simulink model "tf_hex"  (R2020a)
settings: Solver=FixedStepAuto  StartTime=0.0  StopTime=10.0  FixedStep=step_size  RelTol=1e-3
values from neighbouring files (symbols this model uses):
  A = diag([Ax Ax Ax])    [tf_model_sim.m]
  g = 9.81    [tf_model_sim.m]
  m = 1.89    [tf_model_sim.m]
  pitch_tf = tf([omega_n^2], [1 2*zeta*omega_n omega_n^2])*tf([pl],[1 pl],'InputDelay',0.09)    [tf_model_sim.m]
  Ts = 0.01    [tf_model_sim.m]
settings Model: Creator=pala  LastModifiedBy=pala
settings DataIOCC: SaveFormat=StructureWithTime  ReturnWorkspaceOutputs=off

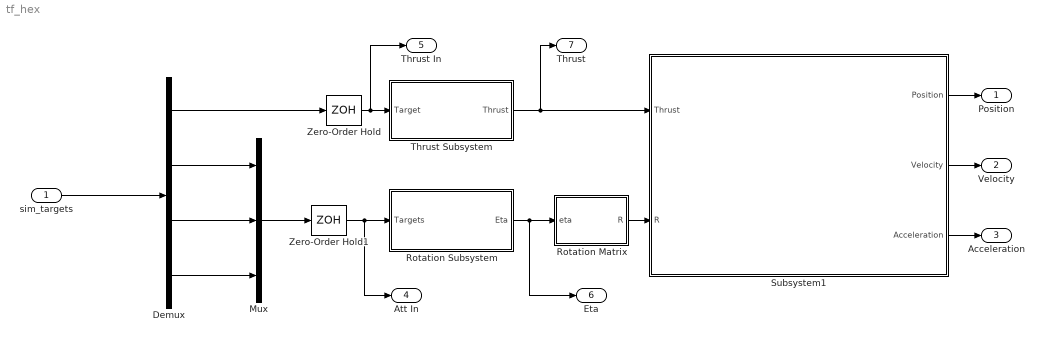
== system tf_hex ==
  sim_targets : Inport
  Demux : Demux
  Mux : Mux  Inputs=3
  Rotation Matrix : MATLAB Function  TreatAsAtomicUnit=on
  Rotation Subsystem : Subsystem
  Subsystem1 : Subsystem
  Thrust Subsystem : Subsystem
  Zero-Order Hold : ZeroOrderHold  SampleTime=Ts
  Zero-Order Hold1 : ZeroOrderHold  SampleTime=Ts
  Position : Outport
  Velocity : Outport  Port=2
  Acceleration : Outport  Port=3
  Att In : Outport  Port=4
  Thrust In : Outport  Port=5
  Eta : Outport  Port=6
  Thrust : Outport  Port=7
  wires:
  sim_targets/1 -> Demux/1
  Demux/2 -> Mux/1
  Demux/3 -> Mux/2
  Demux/4 -> Mux/3
  Subsystem1/2(Velocity) -> Velocity/1
  Subsystem1/3(Acceleration) -> Acceleration/1
  Thrust Subsystem/1(Thrust) -> Thrust/1, Subsystem1/1(Thrust)
  Subsystem1/1(Position) -> Position/1
  Rotation Matrix/1(R) -> Subsystem1/2(R)
  Zero-Order Hold/1 -> Thrust In/1, Thrust Subsystem/1(Target)
  Demux/1 -> Zero-Order Hold/1
  Mux/1 -> Zero-Order Hold1/1
  Zero-Order Hold1/1 -> Att In/1, Rotation Subsystem/1(Targets)
  Rotation Subsystem/1(Eta) -> Eta/1, Rotation Matrix/1(eta)

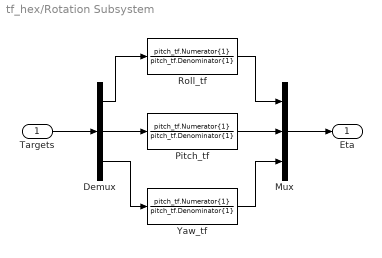
== system tf_hex/Rotation Subsystem ==
  Targets : Inport
  Demux : Demux  Outputs=3
  Mux : Mux  Inputs=3
  Pitch_tf : TransferFcn  Numerator=pitch_tf.Numerator{1}  Denominator=pitch_tf.Denominator{1}
  Roll_tf : TransferFcn  Numerator=pitch_tf.Numerator{1}  Denominator=pitch_tf.Denominator{1}
  Yaw_tf : TransferFcn  Numerator=pitch_tf.Numerator{1}  Denominator=pitch_tf.Denominator{1}
  Eta : Outport
  wires:
  Demux/1 -> Roll_tf/1
  Demux/2 -> Pitch_tf/1
  Demux/3 -> Yaw_tf/1
  Targets/1 -> Demux/1
  Pitch_tf/1 -> Mux/2
  Roll_tf/1 -> Mux/1
  Yaw_tf/1 -> Mux/3
  Mux/1 -> Eta/1

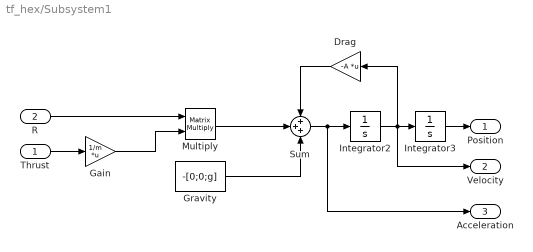
== system tf_hex/Subsystem1 ==
  Thrust : Inport
  R : Inport  Port=2
  Drag : Gain  Gain=-A  Multiplication=Matrix(K*u)
  Gain : Gain  Gain=1/m  Multiplication=Matrix(K*u)
  Gravity : Constant  Value=-[0;0;g]
  Integrator2 : Integrator
  Integrator3 : Integrator
  Multiply : Product  Inputs=**  Multiplication=Matrix(*)
  Sum : Sum  Inputs=+++
  Position : Outport  VectorParamsAs1DForOutWhenUnconnected=off
  Velocity : Outport  Port=2  VectorParamsAs1DForOutWhenUnconnected=off
  Acceleration : Outport  Port=3  VectorParamsAs1DForOutWhenUnconnected=off
  wires:
  Sum/1 -> Acceleration/1, Integrator2/1
  R/1 -> Multiply/1
  Gravity/1 -> Sum/3
  Thrust/1 -> Gain/1
  Integrator3/1 -> Position/1
  Integrator2/1 -> Drag/1, Velocity/1, Integrator3/1
  Multiply/1 -> Sum/2
  Gain/1 -> Multiply/2
  Drag/1 -> Sum/1

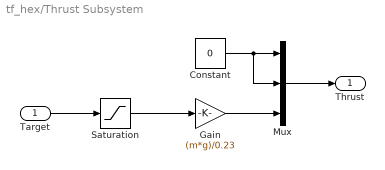
== system tf_hex/Thrust Subsystem ==
  Target : Inport
  Constant : Constant  Value=0
  Gain : Gain  Gain=(m*g)/0.23
  Mux : Mux  Inputs=3
  Saturation : Saturate  UpperLimit=1  LowerLimit=0
  Thrust : Outport
  wires:
  Saturation/1 -> Gain/1
  Target/1 -> Saturation/1
  Constant/1 -> Mux/2, Mux/1
  Mux/1 -> Thrust/1
  Gain/1 -> Mux/3

== matlab function tf_hex/Rotation Matrix ==
  data: eta input; R output
function R = fcn(eta)
eta_deg = rad2deg(eta);
phi     = eta_deg(1);
theta   = eta_deg(2);
psi     = eta_deg(3);

Rz = rotz(psi);
Ry = roty(theta);
Rx = rotx(phi);

R = Rz*Ry*Rx;
